simulink model "SimpleModel"  (R2018b)
settings: Solver=VariableStepAuto  StartTime=0.0  StopTime=10.0  RelTol=1e-3
libraries: simulink x4, UWSimulink3DAnimationBlockset x2, simulink_extras x1, aerolibanimutils x1, vrlib x1
settings Model: Creator=Christopher  LastModifiedBy=chris

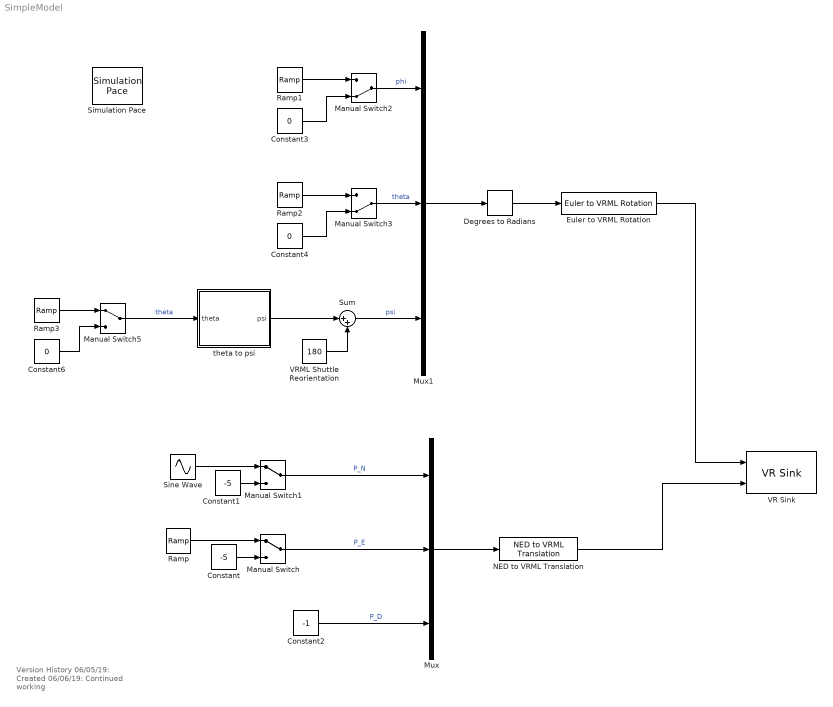
== system SimpleModel ==
  note: Version History
      | 06/05/19: Created
      | 06/06/19: Continued working
  Constant : Constant  Value=-5
  Constant1 : Constant  Value=-5
  Constant2 : Constant  Value=-1
  Constant3 : Constant  Value=0
  Constant4 : Constant  Value=0
  Constant6 : Constant  Value=0
  Degrees to Radians : simulink_extras/Transformations/Degrees to Radians
  Euler to VRML Rotation : UWSimulink3DAnimationBlockset/Euler to VRML Rotation
  Manual Switch : ManualSwitch
  Manual Switch1 : ManualSwitch
  Manual Switch2 : ManualSwitch  CurrentSetting=0
  Manual Switch3 : ManualSwitch  CurrentSetting=0
  Manual Switch5 : ManualSwitch
  Mux : Mux  Inputs=3
  Mux1 : Mux  Inputs=3
  NED to VRML Translation : UWSimulink3DAnimationBlockset/NED to VRML Translation
  Ramp : simulink/Sources/Ramp  slope=1  start=0  InitialOutput=0
  Ramp1 : simulink/Sources/Ramp  slope=30  start=0  InitialOutput=0
  Ramp2 : simulink/Sources/Ramp  slope=30  start=0  InitialOutput=0
  Ramp3 : simulink/Sources/Ramp  slope=30  start=0  InitialOutput=0
  Simulation Pace : aerolibanimutils/Simulation Pace  SimulationPace=1  SleepMode=Auto  OutputPaceError=off  SampleTime=1/30
  Sine Wave : Sin  SampleTime=0
  Sum : Sum  Inputs=|++
  VR Sink : vrlib/VR Sink  InstantiateOnLoad=on  SampleTime=0.1  ViewEnable=on  RemoteChange=off  RemoteView=off  FieldsWritten=Shuttle.rotation.4.1.1.double#Shuttle.translation.3.1.1.double  WorldFileName=CoordinateSystem.wrl  AutoView=on  VideoDimensions=[]  AllowVariableSize=off  FigureProperties="{'Position', 'Name', 'Viewpoint', 'CameraBound', 'CameraDirection', 'CameraPosition', 'CameraUpVector', 'ZoomFactor', 'Antialiasing', 'Headlight', 'Lighting', 'NavPanel', 'Sound', 'StatusBar', 'Stereo3D', 'Stereo3DCameraOffset', 'Stereo3DHIT', 'ToolBar', 'Textures', 'Transparency', 'Triad', 'Wireframe', 'NavZones', 'NavMode', 'NavSpeed', 'CaptureFileFormat', 'CaptureFileName', 'Record2DCompressMethod', 'Record2DCompressQuality', 'Record2D', 'Record2DFileName', 'Record2DFPS'; [-1.5990000000000000e+03   4.2500000000000011e+02   1.6000000000000000e+03   7.7733333333333326e+02], '', 'TopView', 'on', [0.0000000000000000e+00   0.0000000000000000e+00  -1.0000000000000000e+00], [0.0000000000000000e+00   0.0000000000000000e+00   0.0000000000000000e+00], [0.0000000000000000e+00   1.0000000000000000e+00   0.0000000000000000e+00], [1.0000000000000000e+00], 'on', 'on', 'on', 'halfbar', 'on', 'on', 'off', [1.0000000149011612e-01], [0.0000000000000000e+00], 'on', 'on', 'on', 'none', 'off', 'off', 'fly', 'normal', 'tif', '%f_anim_%n.tif', 'auto', [7.5000000000000000e+01], 'off', '%f_anim_%n.avi', 'auto'}"
      settings: SourceProductBaseCode=VR
  VRML Shuttle Reorientation : Constant  Value=180
  theta to psi : Subsystem
  wires:
  Ramp/1 -> Manual Switch/1
  Sine Wave/1 -> Manual Switch1/1
  Constant/1 -> Manual Switch/2
  Constant1/1 -> Manual Switch1/2
  Constant2/1 -> Mux/3  "P_D"
  Mux/1 -> NED to VRML Translation/1
  Manual Switch1/1 -> Mux/1  "P_N"
  Manual Switch/1 -> Mux/2  "P_E"
  NED to VRML Translation/1 -> VR Sink/2
  Mux1/1 -> Degrees to Radians/1
  Ramp1/1 -> Manual Switch2/1
  Manual Switch2/1 -> Mux1/1  "phi"
  Constant3/1 -> Manual Switch2/2
  Degrees to Radians/1 -> Euler to VRML Rotation/1
  Constant4/1 -> Manual Switch3/2
  Ramp2/1 -> Manual Switch3/1
  Manual Switch3/1 -> Mux1/2  "theta"
  theta to psi/1(psi) -> Sum/1
  Sum/1 -> Mux1/3  "psi"
  Euler to VRML Rotation/1 -> VR Sink/1
  Manual Switch5/1 -> theta to psi/1(theta)  "theta"
  VRML Shuttle Reorientation/1 -> Sum/2
  Ramp3/1 -> Manual Switch5/1
  Constant6/1 -> Manual Switch5/2

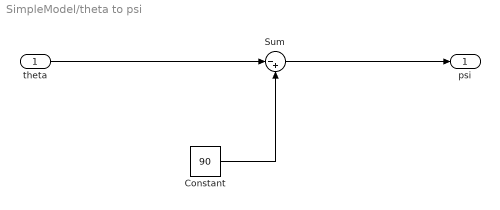
== system SimpleModel/theta to psi ==
  theta : Inport
  Constant : Constant  Value=90
  Sum : Sum  Inputs=|-+
  psi : Outport
  wires:
  theta/1 -> Sum/1
  Constant/1 -> Sum/2
  Sum/1 -> psi/1
